simulink model "model_locreg"  (R2021b)
settings: Solver=VariableStepAuto  StartTime=0.0  StopTime=10  RelTol=1e-3
undefined symbols (not defined in the file): K, Kack
libraries: dsparch4 x1, simulink x1
settings Model: Creator=mateusz  LastModifiedBy=mateusz

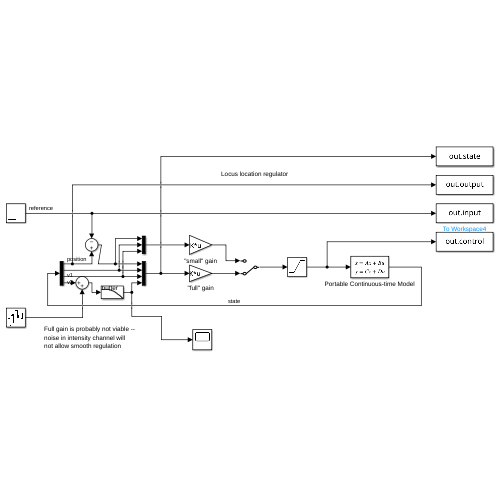
[thumbnail: Simulink's stored preview of the top-level diagram]
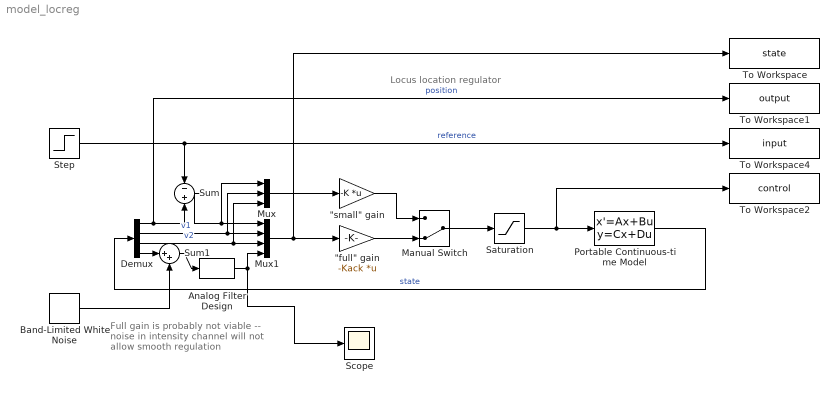
== system model_locreg ==
  note: Full gain is probably not viable -- noise in intensity channel will not allow smooth regulation
  note: Locus location regulator
  "\"full\" gain" : Gain  Gain=-Kack  Multiplication=Matrix(K*u)
  "\"small\" gain" : Gain  Gain=-K  Multiplication=Matrix(K*u)
  Analog Filter Design : dsparch4/Analog Filter Design  method=Butterworth  filttype=Lowpass  N=1  Wlo=6.28*2000  Whi=80  Rp=2  Rs=40
  Band-Limited White Noise : simulink/Sources/Band-Limited White Noise  Cov=[0.0001]  Ts=0.02  seed=[23341]
  Demux : Demux
  Manual Switch : ManualSwitch  CurrentSetting=0
  Mux : Mux  Inputs=3
  Mux1 : Mux
  Portable Continuous-time Model : StateSpace  A=|  B=[0;0;0;2.59e4];  C=eye(4,4)  D=zeros(4,1)  InitialCondition=0
      | [0  1  0    0;
      |      0 -5  4.5  0;
      |      0  0 -0.7108*2  2*23.6012;
      |      0  0 -5.3898 -4040];
  Saturation : Saturate  UpperLimit=.5  LowerLimit=-.5
  Scope : Scope
  Step : Step  After=6.28*25  SampleTime=0
  Sum : Sum  Inputs=-|+
  Sum1 : Sum  Inputs=|++
  To Workspace : ToWorkspace  VariableName=state  SampleTime=-1
  To Workspace1 : ToWorkspace  VariableName=output  SampleTime=-1
  To Workspace2 : ToWorkspace  VariableName=control  SaveFormat=Structure With Time  SampleTime=0.001
  To Workspace4 : ToWorkspace  VariableName=input  SaveFormat=Structure With Time  SampleTime=-1
  wires:
  Step/1 -> Sum/1, To Workspace4/1  "reference"
  Mux/1 -> "\"small\" gain"/1
  Saturation/1 -> Portable Continuous-time Model/1, To Workspace2/1
  Portable Continuous-time Model/1 -> Demux/1  "state"
  Demux/3 -> Mux/3, Mux1/3  "v2"
  Demux/2 -> Mux/2, Mux1/2  "v1"
  Demux/1 -> To Workspace1/1, Sum/2  "position"
  Sum/1 -> Mux/1, Mux1/1
  Manual Switch/1 -> Saturation/1
  Mux1/1 -> To Workspace/1, "\"full\" gain"/1
  "\"small\" gain"/1 -> Manual Switch/1
  "\"full\" gain"/1 -> Manual Switch/2
  Demux/4 -> Sum1/1
  Band-Limited White Noise/1 -> Sum1/2
  Sum1/1 -> Analog Filter Design/1
  Analog Filter Design/1 -> Scope/1, Mux1/4
